simulink subsystem "rollover_handler"  (R2022b)
settings: Solver=VariableStepAuto  StartTime=0.0  StopTime=0.0025  RelTol=1e-3
settings Model: DefaultTestHarness=rollover_handler_harness  Creator=andre  LastModifiedBy=andre
settings ModelReferenceCC: EnableRefExpFcnMdlSchedulingChecks=on

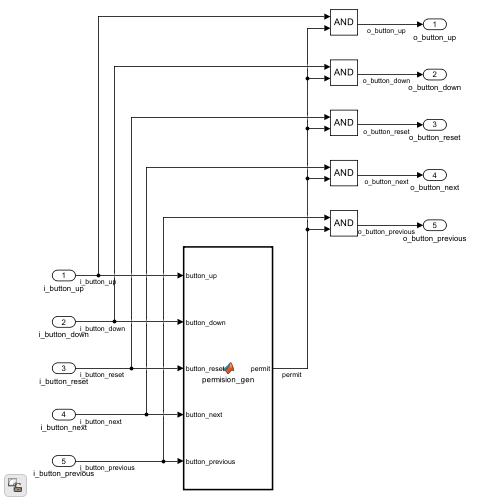
[thumbnail: Simulink's stored preview of the top-level diagram]
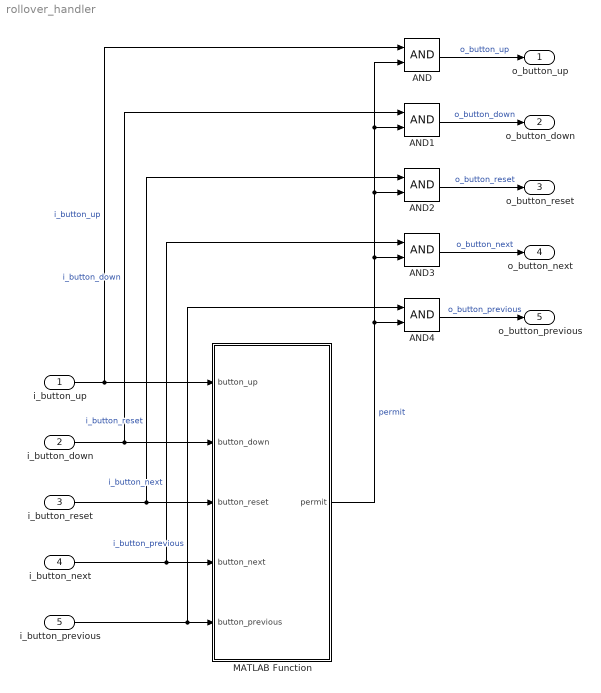
== system rollover_handler ==
  i_button_up : Inport  OutDataTypeStr=boolean  PortDimensions=1
  i_button_down : Inport  Port=2  OutDataTypeStr=boolean  PortDimensions=1
  i_button_reset : Inport  Port=3  OutDataTypeStr=boolean  PortDimensions=1
  i_button_next : Inport  Port=4  OutDataTypeStr=boolean  PortDimensions=1
  i_button_previous : Inport  Port=5  OutDataTypeStr=boolean  PortDimensions=1
  AND{,1..4} (5 alike) : Logic  AllPortsSameDT=off  OutDataTypeStr=boolean
  MATLAB Function : MATLAB Function  TreatAsAtomicUnit=on
  o_button_up : Outport  OutDataTypeStr=boolean  PortDimensions=1
  o_button_down : Outport  Port=2  OutDataTypeStr=boolean  PortDimensions=1
  o_button_reset : Outport  Port=3  OutDataTypeStr=boolean  PortDimensions=1
  o_button_next : Outport  Port=4  OutDataTypeStr=boolean  PortDimensions=1
  o_button_previous : Outport  Port=5  OutDataTypeStr=boolean  PortDimensions=1
  wires:
  MATLAB Function/1(permit) -> AND/2, AND1/2, AND2/2, AND3/2, AND4/2  "permit"
  AND4/1 -> o_button_previous/1  "o_button_previous"
  AND3/1 -> o_button_next/1  "o_button_next"
  AND2/1 -> o_button_reset/1  "o_button_reset"
  AND1/1 -> o_button_down/1  "o_button_down"
  AND/1 -> o_button_up/1  "o_button_up"
  i_button_up/1 -> MATLAB Function/1(button_up), AND/1  "i_button_up"
  i_button_reset/1 -> MATLAB Function/3(button_reset), AND2/1  "i_button_reset"
  i_button_down/1 -> MATLAB Function/2(button_down), AND1/1  "i_button_down"
  i_button_next/1 -> MATLAB Function/4(button_next), AND3/1  "i_button_next"
  i_button_previous/1 -> MATLAB Function/5(button_previous), AND4/1  "i_button_previous"

== matlab function rollover_handler/MATLAB Function ==
  settings: updateMethod=DISCRETE  sampleTime=5e-9
  data: button_up input boolean; permit output boolean; button_down input boolean; button_reset input boolean; button_next input boolean; button_previous input boolean
function permit = permision_gen(button_up, button_down, button_reset, button_next, button_previous)
permit = (~button_up & ~button_down & ~button_reset & ~button_next & button_previous) | ...
         (~button_up & ~button_down & ~button_reset & button_next  & ~button_previous) | ...
         (~button_up & ~button_down & button_reset  & ~button_next & ~button_previous) | ...
         (~button_up & button_down  & ~button_reset & ~button_next & ~button_previous) | ...
         (button_up  & ~button_down & ~button_reset & ~button_next & ~button_previous);
end
